simulink model "Pendulum_sim"  (R2015a)
settings: Solver=ode45  StartTime=0.0  StopTime=10.0  RelTol=1e-3
InitFcn:
  | Ts = 0.02;
  | %SMC Parameters
  | lambda = 1; %surface
  | beta = 200;  %pull magnitude
  | U = 0.01;     %saturation
  | %system parameters
  | m = 15;
  | g = 9.81;
  | L = 1.7;
  | b = 2.0;
  | %system parameter estimates
  | m_hat = 15;
  | g_hat = 9.81;
  | L_hat = 1.7;
  | b_hat = 2.0;
libraries: simulink x1
settings Model: Creator=Logan  LastModifiedBy=Logan

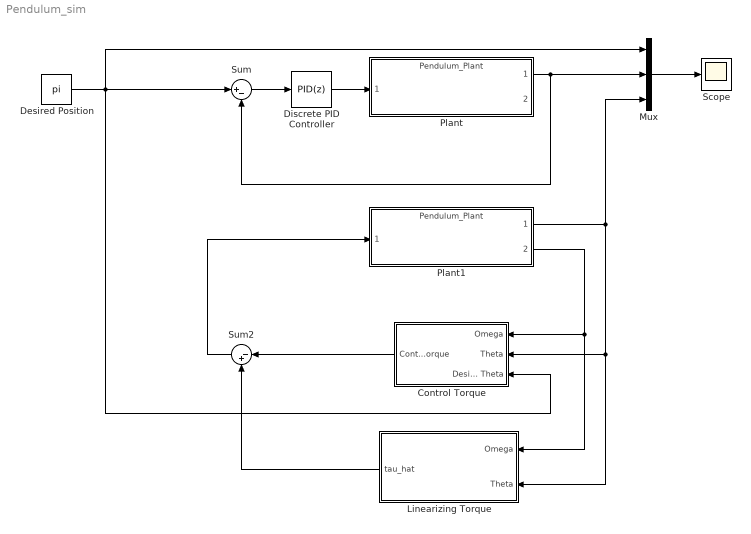
== system Pendulum_sim ==
  Control Torque : Subsystem
  Desired Position : Constant  Value=pi  SampleTime=Ts
  Discrete PID Controller : simulink/Continuous/PID Controller  Controller=PID  TimeDomain=Discrete-time  SampleTime=0.01  IntegratorMethod=Forward Euler  FilterMethod=Forward Euler  Form=Parallel  UseFilter=off  ControllerParametersSource=internal  P=500  I=25  D=250  N=250  InitialConditionSource=internal  InitialConditionForIntegrator=0  InitialConditionForFilter=0  ExternalReset=none  LimitOutput=off  UpperSaturationLimit=inf  LowerSaturationLimit=-inf  LinearizeAsGain=off  AntiWindupMode=none  Kb=1  TrackingMode=off  Kt=1  PParamMin=[]  PParamMax=[]  IParamMin=[]  IParamMax=[]  DParamMin=[]  DParamMax=[]  NParamMin=[]  NParamMax=[]  KbParamMin=[]  KbParamMax=[]  KtParamMin=[]  KtParamMax=[]  POutMin=[]  POutMax=[]  IOutMin=[]  IOutMax=[]  DOutMin=[]  DOutMax=[]  NOutMin=[]  NOutMax=[]  KbOutMin=[]  KbOutMax=[]  KtOutMin=[]  KtOutMax=[]  IntegratorOutMin=[]  IntegratorOutMax=[]  FilterOutMin=[]  FilterOutMax=[]  SumOutMin=[]  SumOutMax=[]  SumI1OutMin=[]  SumI1OutMax=[]  SumI2OutMin=[]  SumI2OutMax=[]  SumI3OutMin=[]  SumI3OutMax=[]  SumDOutMin=[]  SumDOutMax=[]  SaturationOutMin=[]  SaturationOutMax=[]  IntegratorContinuousStateAttributes=''  IntegratorStateMustResolveToSignalObject=off  IntegratorRTWStateStorageClass=Auto  FilterContinuousStateAttributes=''  FilterStateMustResolveToSignalObject=off  FilterRTWStateStorageClass=Auto  DifferentiatorICPrevScaledInput=0  DifferentiatorOutMin=[]  DifferentiatorOutMax=[]
  Linearizing Torque : Subsystem
  Mux : Mux  Inputs=3
  Plant : ModelReference  ModelNameDialog=Pendulum_Plant  SimulationMode=Normal  ModelReferenceVersion=1.40  CopyOfModelName=Pendulum_Plant
  Plant1 : ModelReference  ModelNameDialog=Pendulum_Plant  SimulationMode=Normal  ModelReferenceVersion=1.40  CopyOfModelName=Pendulum_Plant
  Scope : Scope
      settings: TimeRange=10  YMin=0  YMax=3.75
  Sum : Sum  Inputs=|+-
  Sum2 : Sum  Inputs=|-+
  wires:
  Discrete PID Controller/1 -> Plant/1
  Plant/1 -> Mux/2, Sum/2
  Sum/1 -> Discrete PID Controller/1
  Desired Position/1 -> Sum/1, Mux/1, Control Torque/3(Desired Theta)
  Mux/1 -> Scope/1
  Plant1/1 -> Linearizing Torque/2(Theta), Control Torque/2(Theta), Mux/3
  Plant1/2 -> Linearizing Torque/1(Omega), Control Torque/1(Omega)
  Linearizing Torque/1(tau_hat) -> Sum2/2
  Sum2/1 -> Plant1/1
  Control Torque/1(Control Torque) -> Sum2/1

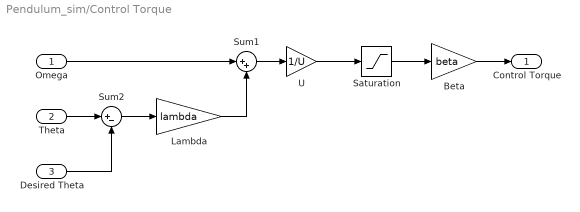
== system Pendulum_sim/Control Torque ==
  Omega : Inport
  Theta : Inport  Port=2
  Desired Theta : Inport  Port=3
  Beta : Gain  Gain=beta
  Lambda : Gain  Gain=lambda
  Saturation : Saturate  UpperLimit=1  LowerLimit=-1
  Sum1 : Sum  Inputs=|++
  Sum2 : Sum  Inputs=|+-
  U : Gain  Gain=1/U
  Control Torque : Outport
  wires:
  Lambda/1 -> Sum1/2
  Omega/1 -> Sum1/1
  Saturation/1 -> Beta/1
  Beta/1 -> Control Torque/1
  Theta/1 -> Sum2/1
  Sum2/1 -> Lambda/1
  Desired Theta/1 -> Sum2/2
  U/1 -> Saturation/1
  Sum1/1 -> U/1

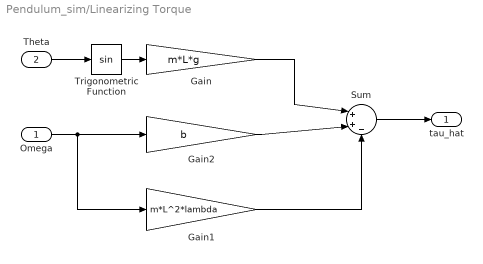
== system Pendulum_sim/Linearizing Torque ==
  Omega : Inport
  Theta : Inport  Port=2
  Gain : Gain  Gain=m*L*g
  Gain1 : Gain  Gain=m*L^2*lambda
  Gain2 : Gain  Gain=b
  Sum : Sum  Inputs=|++-
  Trigonometric Function : Trigonometry
  tau_hat : Outport
  wires:
  Theta/1 -> Trigonometric Function/1
  Trigonometric Function/1 -> Gain/1
  Omega/1 -> Gain1/1, Gain2/1
  Gain/1 -> Sum/1
  Gain2/1 -> Sum/2
  Gain1/1 -> Sum/3
  Sum/1 -> tau_hat/1
